simulink model "PMSM_id_zero"  (R2015a)
settings: Solver=ode45  StartTime=0.0  StopTime=5  RelTol=1e-3
values from neighbouring files (symbols this model uses):
  D = 1    [PMSM_id_zero_config.m]
  J = 1    [PMSM_id_zero_config.m]
  Ld = 0.97e-3    (= 0.00097)    [PMSM_id_zero_config.m]
  Lq = 2.03e-3    (= 0.00203)    [PMSM_id_zero_config.m]
  Phia = Ke    (= 0.0432)    [PMSM_id_zero_config.m]
  Pn = 3    [PMSM_id_zero_config.m]
  R = 0.1197    [PMSM_id_zero_config.m]
settings Model: Creator=hamada  LastModifiedBy=hamada

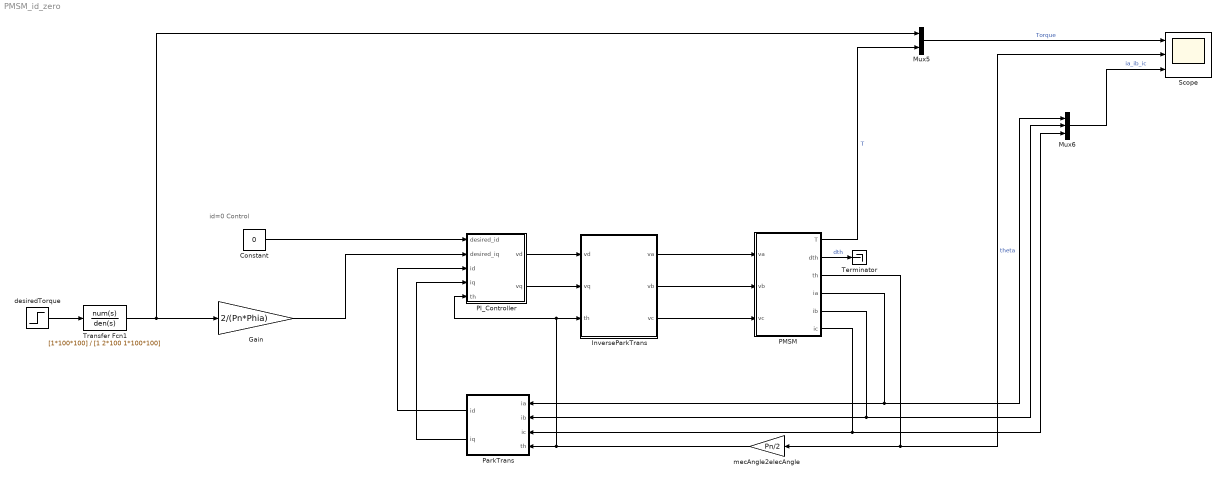
== system PMSM_id_zero ==
  note: id=0 Control
  Constant : Constant  Value=0
  Gain : Gain  Gain=2/(Pn*Phia)
  InverseParkTrans : MATLAB Function  TreatAsAtomicUnit=on  SystemSampleTime=0.001
  Mux5 : Mux  Inputs=2
  Mux6 : Mux  Inputs=3
  PI_Controller : Subsystem  SystemSampleTime=0.001
  PMSM : Subsystem
  ParkTrans : MATLAB Function  TreatAsAtomicUnit=on
  Scope : Scope  NumInputPorts=3
      settings: TimeRange=5  YMin=0~0~-80  YMax=5~15~80
  Terminator : Terminator
  Transfer Fcn1 : TransferFcn  Numerator=[1*100*100]  Denominator=[1 2*100 1*100*100]
  desiredTorque : Step  After=5  SampleTime=0
  mecAngle2elecAngle : Gain  Gain=Pn/2
  wires:
  PMSM/1(T) -> Mux5/2  "T"
  PMSM/3(th) -> Scope/2, mecAngle2elecAngle/1  "theta"
  desiredTorque/1 -> Transfer Fcn1/1
  PMSM/4(ia) -> ParkTrans/1(ia), Mux6/1
  PMSM/5(ib) -> ParkTrans/2(ib), Mux6/2
  PMSM/6(ic) -> ParkTrans/3(ic), Mux6/3
  InverseParkTrans/2(vb) -> PMSM/2(vb)
  InverseParkTrans/3(vc) -> PMSM/3(vc)
  InverseParkTrans/1(va) -> PMSM/1(va)
  Constant/1 -> PI_Controller/1(desired_id)
  Gain/1 -> PI_Controller/2(desired_iq)
  mecAngle2elecAngle/1 -> PI_Controller/5(th), InverseParkTrans/3(th), ParkTrans/4(th)
  Transfer Fcn1/1 -> Mux5/1, Gain/1
  PI_Controller/1(vd) -> InverseParkTrans/1(vd)
  PI_Controller/2(vq) -> InverseParkTrans/2(vq)
  ParkTrans/1(id) -> PI_Controller/3(id)
  ParkTrans/2(iq) -> PI_Controller/4(iq)
  PMSM/2(dth) -> Terminator/1  "dth"
  Mux5/1 -> Scope/1  "Torque"
  Mux6/1 -> Scope/3  "ia_ib_ic"

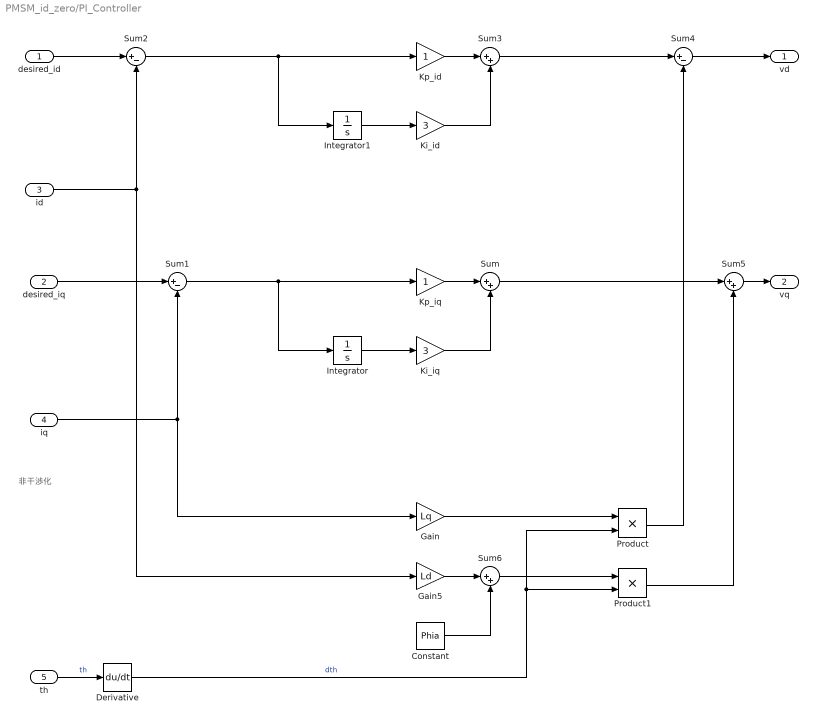
== system PMSM_id_zero/PI_Controller ==
  note: 非干渉化
  desired_id : Inport
  desired_iq : Inport  Port=2
  id : Inport  Port=3
  iq : Inport  Port=4
  th : Inport  Port=5
  Constant : Constant  Value=Phia
  Derivative : Derivative
  Gain : Gain  Gain=Lq
  Gain5 : Gain  Gain=Ld
  Integrator : Integrator
  Integrator1 : Integrator
  Ki_id : Gain  Gain=3
  Ki_iq : Gain  Gain=3
  Kp_id : Gain
  Kp_iq : Gain
  Product : Product
  Product1 : Product
  Sum{,3,5..6} (4 alike) : Sum  Inputs=|++
  Sum1 : Sum  Inputs=|+-
  Sum2 : Sum  Inputs=|+-
  Sum4 : Sum  Inputs=|+-
  vd : Outport
  vq : Outport  Port=2
  wires:
  Sum1/1 -> Integrator/1, Kp_iq/1
  desired_id/1 -> Sum2/1
  Kp_iq/1 -> Sum/1
  desired_iq/1 -> Sum1/1
  id/1 -> Sum2/2, Gain5/1
  iq/1 -> Sum1/2, Gain/1
  Sum/1 -> Sum5/1
  Integrator/1 -> Ki_iq/1
  Ki_iq/1 -> Sum/2
  Sum2/1 -> Integrator1/1, Kp_id/1
  Kp_id/1 -> Sum3/1
  Sum3/1 -> Sum4/1
  Integrator1/1 -> Ki_id/1
  Ki_id/1 -> Sum3/2
  th/1 -> Derivative/1  "th"
  Derivative/1 -> Product/2, Product1/2  "dth"
  Gain/1 -> Product/1
  Product/1 -> Sum4/2
  Sum4/1 -> vd/1
  Sum5/1 -> vq/1
  Gain5/1 -> Sum6/1
  Constant/1 -> Sum6/2
  Sum6/1 -> Product1/1
  Product1/1 -> Sum5/2

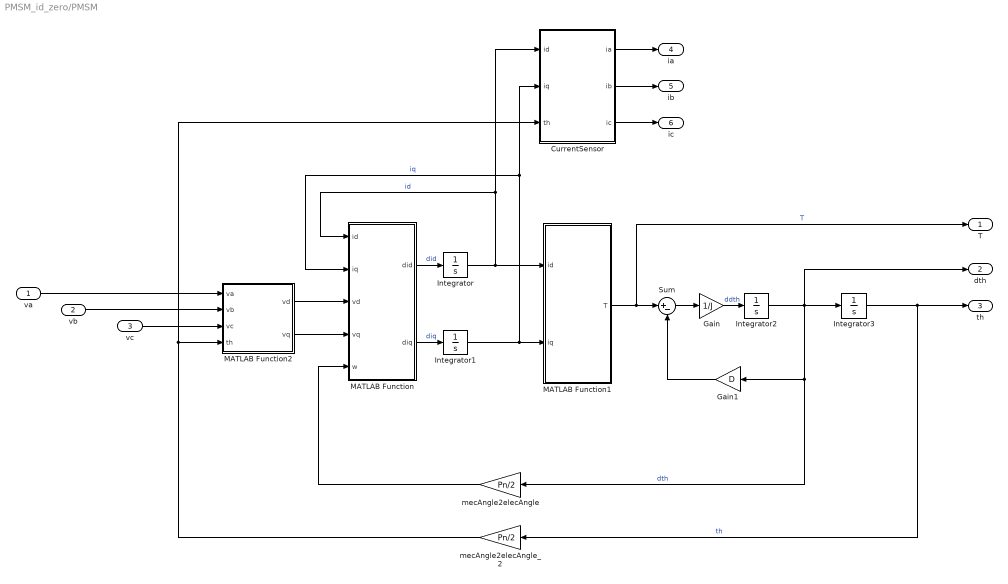
== system PMSM_id_zero/PMSM ==
  va : Inport
  vb : Inport  Port=2
  vc : Inport  Port=3
  CurrentSensor : MATLAB Function  TreatAsAtomicUnit=on
  Gain : Gain  Gain=1/J
  Gain1 : Gain  Gain=D
  Integrator{,1..3} (4 alike) : Integrator
  MATLAB Function : MATLAB Function  TreatAsAtomicUnit=on
  MATLAB Function1 : MATLAB Function  TreatAsAtomicUnit=on
  MATLAB Function2 : MATLAB Function  TreatAsAtomicUnit=on
  Sum : Sum  Inputs=|+-
  mecAngle2elecAngle : Gain  Gain=Pn/2
  mecAngle2elecAngle_2 : Gain  Gain=Pn/2
  T : Outport
  dth : Outport  Port=2
  th : Outport  Port=3
  ia : Outport  Port=4
  ib : Outport  Port=5
  ic : Outport  Port=6
  wires:
  va/1 -> MATLAB Function2/1(va)
  vb/1 -> MATLAB Function2/2(vb)
  vc/1 -> MATLAB Function2/3(vc)
  MATLAB Function/1(did) -> Integrator/1  "did"
  MATLAB Function/2(diq) -> Integrator1/1  "diq"
  Integrator/1 -> MATLAB Function/1(id), CurrentSensor/1(id), MATLAB Function1/1(id)  "id"
  Integrator1/1 -> MATLAB Function/2(iq), CurrentSensor/2(iq), MATLAB Function1/2(iq)  "iq"
  Sum/1 -> Gain/1
  Gain/1 -> Integrator2/1  "ddth"
  MATLAB Function1/1(T) -> T/1, Sum/1  "T"
  Integrator2/1 -> dth/1, Integrator3/1, mecAngle2elecAngle/1, Gain1/1  "dth"
  Gain1/1 -> Sum/2
  MATLAB Function2/1(vd) -> MATLAB Function/3(vd)
  MATLAB Function2/2(vq) -> MATLAB Function/4(vq)
  Integrator3/1 -> th/1, mecAngle2elecAngle_2/1  "th"
  mecAngle2elecAngle/1 -> MATLAB Function/5(w)
  mecAngle2elecAngle_2/1 -> CurrentSensor/3(th), MATLAB Function2/4(th)
  CurrentSensor/1(ia) -> ia/1
  CurrentSensor/2(ib) -> ib/1
  CurrentSensor/3(ic) -> ic/1

== matlab function PMSM_id_zero/ParkTrans ==
  data: ia input; ib input; ic input; th input; id output; iq output
function [ id, iq ] = fcn( ia, ib, ic, th ) 
    %#codegen
    buff = [
         cos( th ),  cos( th - ( ( 2 * pi ) / 3 ) ),  cos( th + ( ( 2 * pi ) / 3 ) );
        -sin( th ), -sin( th - ( ( 2 * pi ) / 3 ) ), -sin( th + ( ( 2 * pi ) / 3 ) );
        ( 1 / sqrt( 2 ) ), ( 1 / sqrt( 2 ) ), ( 1 / sqrt( 2 ) );
    ];

    idq = sqrt( 2 / 3 ) * buff * [ ia;ib;ic; ];
    id = idq(1);
    iq = idq(2);
end

== matlab function PMSM_id_zero/InverseParkTrans ==
  data: vd input; vq input; va output; vb output; vc output; th input
function [ va, vb, vc ] = fcn( vd, vq, th ) 
    %#codegen
    buff = [
        cos( th ), -sin( th ), ( 1 / sqrt( 2 ) );
        cos( th - ( ( 2 * pi ) / 3 ) ), -sin( th - ( ( 2 * pi ) / 3 ) ), ( 1 / sqrt( 2 ) );
        cos( th + ( ( 2 * pi ) / 3 ) ), -sin( th + ( ( 2 * pi ) / 3 ) ), ( 1 / sqrt( 2 ) );
    ];

    vabc = sqrt( 2 / 3 ) * buff * [ vd;vq;0; ];
    va = vabc(1);
    vb = vabc(2);
    vc = vabc(3);
end

== matlab function PMSM_id_zero/PMSM/MATLAB Function ==
  data: did output; diq output; id input; iq input; vd input; vq input; w input; R parameter; Ld parameter; Lq parameter; Phia parameter
function [ did, diq ] = fcn( id, iq, vd ,vq, w, R, Ld, Lq, Phia ) 
    %#codegen
    
    idq = [ id;iq; ];
    vdq = [ vd;vq; ];
    
    A = [ 
        -( R / Ld ), ( w * ( Lq / Ld ) );
        -( w * ( Ld / Lq ) ), -( R / Lq );
    ];
    
    B = [
        ( 1 / Ld ), 0;
        0, ( 1 / Lq );
    ];

    U = [
        0;
        -( w * ( Phia / Lq ) );
    ];

    didq = A * idq + B * vdq + U;
    
    did = didq(1);
    diq = didq(2);
end

== matlab function PMSM_id_zero/PMSM/MATLAB Function1 ==
  data: T output; id input; iq input; Ld parameter; Lq parameter; Phia parameter; Pn parameter
function T = fcn( id, iq, Ld, Lq, Phia, Pn ) 
    %#codegen
    
    T = ( Pn / 2 ) * ( Phia * iq + ( Ld - Lq ) * id * iq );

end

== matlab function PMSM_id_zero/PMSM/MATLAB Function2 ==
  data: va input; vb input; vc input; th input; vd output; vq output
function [ vd, vq ] = fcn( va, vb, vc, th ) 
    %#codegen
    buff = [
         cos( th ),  cos( th - ( ( 2 * pi ) / 3 ) ),  cos( th + ( ( 2 * pi ) / 3 ) );
        -sin( th ), -sin( th - ( ( 2 * pi ) / 3 ) ), -sin( th + ( ( 2 * pi ) / 3 ) );
        ( 1 / sqrt( 2 ) ), ( 1 / sqrt( 2 ) ), ( 1 / sqrt( 2 ) );
    ];

    vdq = sqrt( 2 / 3 ) * buff * [ va;vb;vc; ];
    vd = vdq(1);
    vq = vdq(2);
end

== matlab function PMSM_id_zero/PMSM/CurrentSensor ==
  data: id input; iq input; ia output; ib output; ic output; th input
function [ ia, ib, ic ] = fcn( id, iq, th ) 
    %#codegen
    buff = [
        cos( th ), -sin( th ), ( 1 / sqrt( 2 ) );
        cos( th - ( ( 2 * pi ) / 3 ) ), -sin( th - ( ( 2 * pi ) / 3 ) ), ( 1 / sqrt( 2 ) );
        cos( th + ( ( 2 * pi ) / 3 ) ), -sin( th + ( ( 2 * pi ) / 3 ) ), ( 1 / sqrt( 2 ) );
    ];

    iabc = sqrt( 2 / 3 ) * buff * [ id;iq;0; ];
    ia = iabc(1);
    ib = iabc(2);
    ic = iabc(3);
end
